simulink model "Stopwatch1"  (Simulink 5.0)
settings: Solver=FixedStepDiscrete  StartTime=0.0  StopTime=100000.0  RelTol=1e-3
libraries: simulink x2
settings Model: Creator=scaife  LastModifiedBy=scaife  ExtModeAutoUpdateStatusClock=off

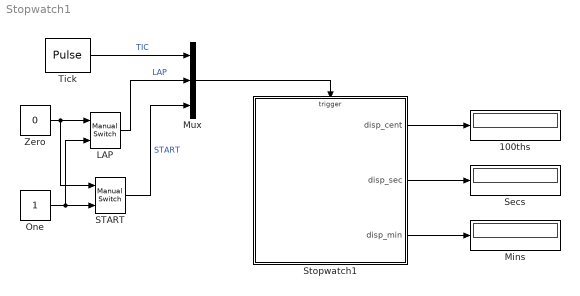
== system Stopwatch1 ==
  100ths : Display
  LAP : simulink/Signal Routing/Manual Switch  sw=1  action=0
  Mins : Display
  Mux : Mux  Inputs=3
  One : Constant
  START : simulink/Signal Routing/Manual Switch  sw=1  action=0
  Secs : Display
  Stopwatch1 : Stateflow chart
  Tick : DiscretePulseGenerator  SampleTime=0.01  VectorParams1D=off
  Zero : Constant  Value=0
  wires:
  Stopwatch1/1(disp_cent) -> 100ths/1
  Stopwatch1/2(disp_sec) -> Secs/1
  Stopwatch1/3(disp_min) -> Mins/1
  Tick/1 -> Mux/1  "TIC"
  Zero/1 -> LAP/1, START/1
  One/1 -> START/2, LAP/2
  LAP/1 -> Mux/2  "LAP"
  Mux/1 -> Stopwatch1/Trigger
  START/1 -> Mux/3  "START"

== stateflow chart Stopwatch1 ==
  state Stopwatch
    state Stop
      state Reset/
        en: runlap=1;
        on LAP:
        cent=0; sec=0; min=0;
        disp_cent=0; disp_sec=0;
        disp_min=0;
      state Lap_stop/
        en: runlap=2;
      (default) -> Reset : [runlap==1]
      (default) -> Lap_stop : [runlap==2]
      Lap_stop -> Reset : LAP
    state Run
      state Watch [parallel]
        state Running/
          en: runlap=1;
          du:
          disp_cent=cent;
          disp_sec=sec;
          disp_min=min;
        state Lap/
          en: runlap=2;
        Running -> Lap : LAP
        Lap -> Running : LAP
        (default) -> Running : [runlap==1]
        (default) -> Lap : [runlap==2]
      state Tick [parallel]
        state TicStart
        TicStart -> (junction 13) : TIC{cent++;}
        (junction 13) -> (junction 14) : [cent==100]{cent=0; sec++;}
        (default) -> TicStart
        (junction 14) -> (junction 15)
        (junction 14) -> (junction 15) : [sec==60]{sec=0; min++;}
        (junction 13) -> (junction 15)
    Stop -> Run : START
    Run -> Stop : START
    (default) -> Stop : {runlap=1;}
  (default) -> Stopwatch
  data: runlap local int32 =1; cent local int32; sec local int32; min local int32; disp_cent output int32; disp_sec output int32; disp_min output int32
  events: TIC input EITHER_EDGE_EVENT; LAP input EITHER_EDGE_EVENT; START input EITHER_EDGE_EVENT
